simulink model "Solar_app_failed"  (R2020a)
settings: Solver=VariableStepAuto  StartTime=0.0  StopTime=10.0  RelTol=1e-3
libraries: powerlib x15, simulink x2, re_lib x1, powerlib_meascontrol x1, powerlib_extras x1
settings Model: Creator=royde  LastModifiedBy=royde

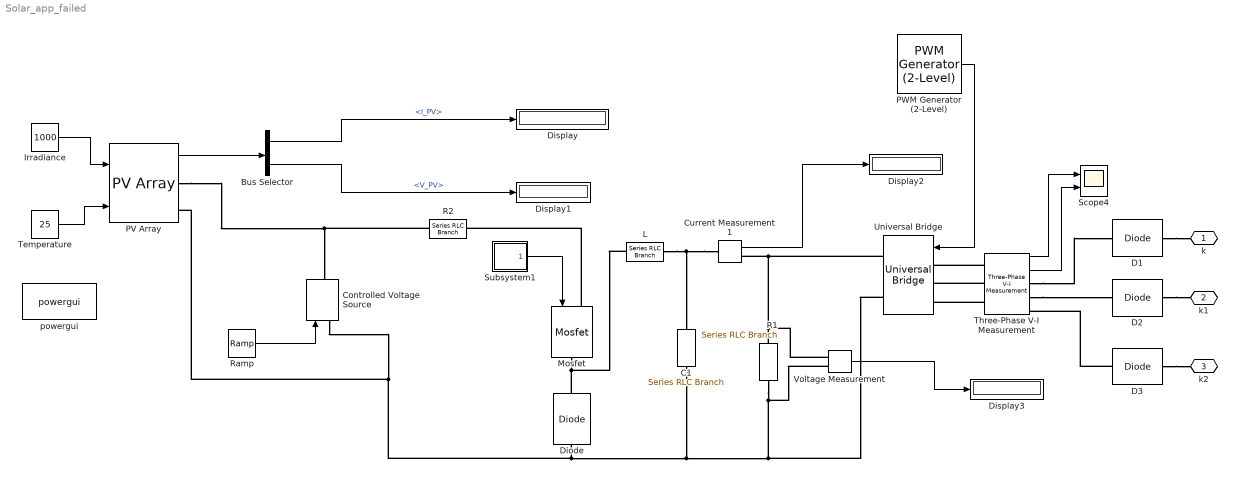
== system Solar_app_failed ==
  Bus Selector : BusSelector  OutputSignals=I_PV,V_PV
  C1 : powerlib/Elements/Series RLC Branch  LConnTagsString=__new0  RConnTagsString=__new0  BranchType=C  Resistance=1  Inductance=1e-3  SetiL0=off  InitialCurrent=0  Capacitance=5000e-6  Setx0=off  InitialVoltage=24  Measurements=Branch voltage and current
  Controlled Voltage Source : powerlib/Electrical Sources/Controlled Voltage Source  Initialize=on  Source_Type=AC  Amplitude=0  Phase=0  Frequency=0  Measurements=None
  Current Measurement1 : powerlib/Measurements/Current Measurement  PhasorSimulation=off  OutputType=Complex  PSBequivalent=0
  D1 : powerlib/Power Electronics/Diode  Ron=0.001  Lon=0  Vf=0.1  IC=0  UseSnubber=off  Rs=50000  Cs=250e-12  Measurements=off
  D2 : powerlib/Power Electronics/Diode  Ron=0.001  Lon=0  Vf=0.1  IC=0  UseSnubber=off  Rs=50000  Cs=250e-12  Measurements=off
  D3 : powerlib/Power Electronics/Diode  Ron=0.001  Lon=0  Vf=0.1  IC=0  UseSnubber=off  Rs=50000  Cs=250e-12  Measurements=off
  Diode : powerlib/Power Electronics/Diode  Ron=0.001  Lon=0  Vf=0.8  IC=0  UseSnubber=off  Rs=500  Cs=250e-9  Measurements=off
  Display{,1..3} (4 alike) : Display
  Irradiance : Constant  Value=1000
  L : powerlib/Elements/Series RLC Branch  LConnTagsString=__new0  RConnTagsString=__new0  BranchType=RL  Resistance=2  Inductance=550e-6  SetiL0=off  InitialCurrent=0  Capacitance=560e-6  Setx0=off  InitialVoltage=0  Measurements=Branch current
  Mosfet : powerlib/Power Electronics/Mosfet  Ron=0.1  Lon=0  Rd=0.01  Vfd=0  IC=0  Rs=1e5  Cs=inf  Measurements=off
  PV Array : re_lib/Solar/PV Array  Npar=3  Nser=3  PlotType=array @ 1000 W/m2 & specified temperatures  S_vec="[ 1000  500  100 ]"  Temp_C_vec="[ 45 25  ]"  ModuleName=SunPower SER-220P  PlotWhenSelected=off  Pm=219.9716  Ncell=60  Voc=36.3  Isc=8.3  Vm=29.02  Im=7.58  beta_Voc_pc=-0.35501  alpha_Isc_pc=0.043795  beta_Voc=-0.12887  alpha_Isc=0.003635  IL=8.3331  I0=2.2787e-10  nI=0.97003  Rsh=95.1262  Rs=0.37924  RobustModel=off  RobustCellTemperature=25  BAL=on  Tc=1e-6  Tfilter=5e-5
  PWM Generator (2-Level) : powerlib_meascontrol/Pulse & Signal Generators/PWM Generator (2-Level)  ModulatorType=Three-phase bridge (6 pulses)  ModulatorMode=Unsynchronized  Fc=27*60  Pc=90  nF=27  MinMax="[ -1  1 ]"  SamplingTechnique=Natural  ModulatingSignals=off  m=0.8  Freq=60  Phase=0  Ts=0  ShowCarrierOutport=off
  R1 : powerlib/Elements/Series RLC Branch  LConnTagsString=__new0  RConnTagsString=__new0  BranchType=R  Resistance=11  Inductance=550e-6  SetiL0=off  InitialCurrent=0  Capacitance=560e-6  Setx0=off  InitialVoltage=0  Measurements=Branch current
  R2 : powerlib/Elements/Series RLC Branch  LConnTagsString=__new0  RConnTagsString=__new0  BranchType=R  Resistance=0.5  Inductance=1e-3  SetiL0=off  InitialCurrent=0  Capacitance=560e-6  Setx0=off  InitialVoltage=0  Measurements=None
  Ramp : simulink/Sources/Ramp  slope=96  start=0  InitialOutput=0
  Scope4 : Scope  NumInputPorts=2
  Subsystem1 : Subsystem
  Temperature : Constant  Value=25
  Three-Phase V-I Measurement : powerlib/Measurements/Three-Phase V-I Measurement  VoltageMeasurement=phase-to-ground  SetLabelV=off  LabelV=Vabc  Vpu=off  VpuLL=off  CurrentMeasurement=yes  SetLabelI=off  LabelI=Iabc  Ipu=off  Pbase=100e6  Vbase=500e3  OutputType=Complex  PhasorSimulation=off  PSBequivalent=0
  Universal Bridge : powerlib/Power Electronics/Universal Bridge  Arms=3  SnubberResistance=1e5  SnubberCapacitance=inf  Device=MOSFET / Diodes  Ron=1e-3  Lon=0  ForwardVoltages="[  0  0  ]"  ForwardVoltage=0  GTOparameters=[ 10e-6 , 20e-6 ]  IGBTparameters=[ 1e-6 , 2e-6 ]  Measurements=None  Measurements_2=None  converterType=Rectifier
  Voltage Measurement : powerlib/Measurements/Voltage Measurement  PhasorSimulation=off  OutputType=Complex  PSBequivalent=0
  powergui : powerlib/powergui  Priority=1  SimulationMode=Continuous  SampleTime=50e-6  frequency=60  Iterations=50  frequencyindice=0  Pbase=100e6  ErrMax=1e-4  UnitsV=kV  UnitsW=MW  buscounter=0  FunctionMessages=off  echomessages=off  EnableUseOfTLC=off  CurrentSourceSwitches=off  DisableSnubberDevices=off  DisableRonSwitches=off  DisableVfSwitches=off  DisplayEquations=off  AutomaticDiscreteSolvers=off  SolverType=Tustin/Backward Euler (TBE)  Interpol=off  ExternalGateDelay=off  methode=off  Ts=100  x0status=blocks  SPID=on  SwTol=0  HookPort=off  NonlinearTolerance=1e-4  nMaxIteration=100  ContinueOnMaxIteration=off  RestoreLinks=warning  ResistiveCurrentMeasurement=off  Frange=[0:2:500]  Ylog=off  Xlog=on  ShowGrid=off  save=off  variable=ZData  structure=0  ZoomFFT=off  StartTime=0.0  cycles=1  DisplayStyle=1  fundamental=60  FreqAxis=off  MaxFrequency=1000  frequencyindicesteady=1  RmsSteady=1  display=off
  k : PMIOPort  Side=Right
  k1 : PMIOPort  Port=2  Side=Right
  k2 : PMIOPort  Port=3  Side=Right
  wires:
  Voltage Measurement/1 -> Display3/1
  Ramp/1 -> Controlled Voltage Source/1
  PV Array/1 -> Bus Selector/1
  Subsystem1/1(Out1) -> Mosfet/1
  Three-Phase V-I Measurement/2 -> Scope4/2
  Irradiance/1 -> PV Array/1
  Bus Selector/1 -> Display/1  "<I_PV>"
  Bus Selector/2 -> Display1/1  "<V_PV>"
  Temperature/1 -> PV Array/2
  Current Measurement1/1 -> Display2/1
  Three-Phase V-I Measurement/1 -> Scope4/1
  PWM Generator (2-Level)/1 -> Universal Bridge/1
  connections:
  Diode/RConn1 -- Mosfet/RConn1 -- L/RConn1
  R1/LConn1 -- Voltage Measurement/LConn2 -- Universal Bridge/RConn2 -- Controlled Voltage Source/LConn1 -- PV Array/RConn2 -- Diode/LConn1 -- C1/RConn1
  R2/RConn1 -- PV Array/RConn1 -- Controlled Voltage Source/RConn1
  Current Measurement1/LConn1 -- L/LConn1 -- C1/LConn1
  Current Measurement1/RConn1 -- R1/RConn1 -- Voltage Measurement/LConn1 -- Universal Bridge/RConn1
  D2/RConn1 -- k1/RConn1
  D3/RConn1 -- k2/RConn1
  D3/LConn1 -- Three-Phase V-I Measurement/RConn3
  Three-Phase V-I Measurement/LConn1 -- Universal Bridge/LConn1
  Three-Phase V-I Measurement/LConn2 -- Universal Bridge/LConn2
  D1/RConn1 -- k/RConn1
  Three-Phase V-I Measurement/LConn3 -- Universal Bridge/LConn3
  Three-Phase V-I Measurement/RConn2 -- D2/LConn1
  Three-Phase V-I Measurement/RConn1 -- D1/LConn1
  Mosfet/LConn1 -- R2/LConn1

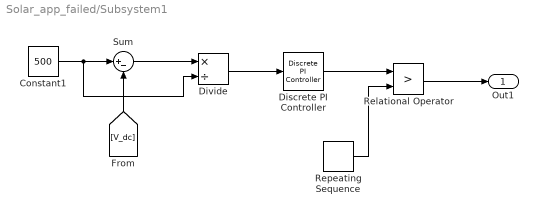
== system Solar_app_failed/Subsystem1 ==
  Constant1 : Constant  Value=500  VectorParams1D=off
  Discrete PI Controller : powerlib_extras/Discrete  Control Blocks/Discrete PI Controller  Kp=10  Ki=78  Par_Limits=[0.99 0]  Init=0.1  Ts=3.3e-6
  Divide : Product  Inputs=*/  SampleTime=3.3e-6
  Relational Operator : RelationalOperator  Operator=>  OutDataTypeStr=boolean  RndMeth=Nearest
  Repeating Sequence : simulink/Sources/Repeating Sequence  rep_seq_t=[0 1/30000]  rep_seq_y="[0  1]"
  Sum : Sum  Inputs=|+-
  Out1 : Outport
  wires:
  Constant1/1 -> Sum/1, Divide/2
  [V_dc] -> Sum/2
  Sum/1 -> Divide/1
  Divide/1 -> Discrete PI Controller/1
  Discrete PI Controller/1 -> Relational Operator/1
  Repeating Sequence/1 -> Relational Operator/2
  Relational Operator/1 -> Out1/1
